simulink model "UV_Model_TT"  (R2020a)
settings: Solver=FixedStepAuto  StartTime=0.0  StopTime=100  FixedStep=0.01  RelTol=1e-3
InitFcn:
  | UV_Parameters;
values from neighbouring files (symbols this model uses):
  KP = 1    [UV_Parameters.m]
  KR = 1    [UV_Parameters.m]
  p0 = [0,0,0]    [UV_Parameters.m]
  R0 = [cos(psi0)*cos(theta0) -sin(psi0)*cos(theta0)+cos(psi0)*sin(theta0)*sin(phi0) sin(psi0)*sin(phi0)+cos(psi0)*sin(theta0)*cos(phi0);        sin(psi0)*cos(theta0) cos(psi0)*cos(theta0)+sin(psi0)*sin(theta0)*sin(phi0)  -cos(psi0)*sin(phi0)+sin(psi0)*sin(theta0)*cos(phi0);        -sin(theta0)  cos(theta0)*sin(phi0)  cos(theta0)*cos(phi0)]    [UV_Parameters.m]
libraries: vrlib x3
settings Model: Creator=vcichella  LastModifiedBy=vcichella
settings SFSimCC: CustomCodeUndefinedFunction=UseInterfaceOnly

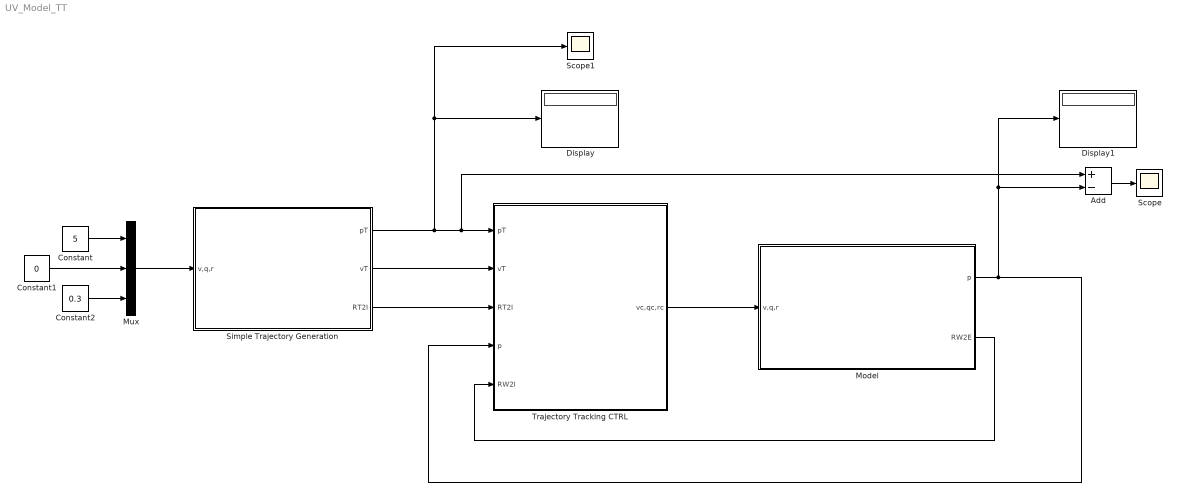
== system UV_Model_TT ==
  Add : Sum  Inputs=+-
  Constant : Constant  Value=5
  Constant1 : Constant  Value=0
  Constant2 : Constant  Value=0.3
  Display : Display
  Display1 : Display
  Model : Subsystem
  Mux : Mux  Inputs=3
  Scope : Scope
  Scope1 : Scope
  Simple Trajectory Generation : Subsystem
  "Trajectory Tracking CTRL " : Subsystem
  wires:
  Simple Trajectory Generation/3(RT2I) -> "Trajectory Tracking CTRL "/3(RT2I)
  Constant/1 -> Mux/1
  Simple Trajectory Generation/1(pT) -> Add/1, "Trajectory Tracking CTRL "/1(pT), Scope1/1, Display/1
  Mux/1 -> Simple Trajectory Generation/1(v,q,r)
  Constant1/1 -> Mux/2
  Constant2/1 -> Mux/3
  Simple Trajectory Generation/2(vT) -> "Trajectory Tracking CTRL "/2(vT)
  Add/1 -> Scope/1
  "Trajectory Tracking CTRL "/1(vc,qc,rc) -> Model/1(v,q,r)
  Model/2(RW2E) -> "Trajectory Tracking CTRL "/5(RW2I)
  Model/1(p) -> "Trajectory Tracking CTRL "/4(p), Add/2, Display1/1

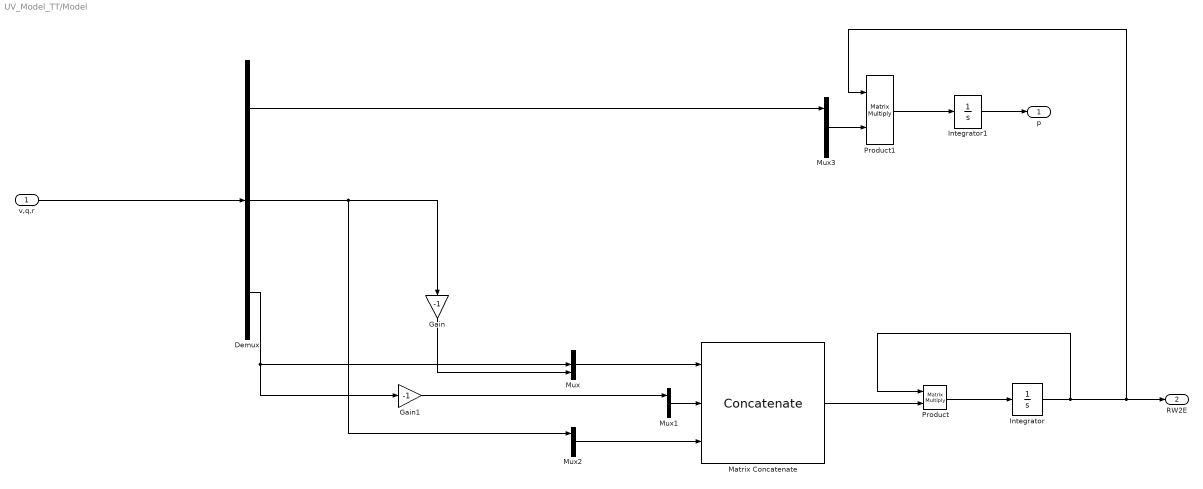
== system UV_Model_TT/Model ==
  v,q,r : Inport
  Demux : Demux  Outputs=3
  Gain : Gain  Gain=-1
  Gain1 : Gain  Gain=-1
  Integrator : Integrator  InitialCondition=R0
  Integrator1 : Integrator  InitialCondition=p0
  Matrix Concatenate : Concatenate  NumInputs=3  Mode=Multidimensional array  ConcatenateDimension=2
  Mux{,1..3} (4 alike) : Mux  Inputs=3
  Product : Product  Multiplication=Matrix(*)
  Product1 : Product  Multiplication=Matrix(*)
  p : Outport  VectorParamsAs1DForOutWhenUnconnected=off
  RW2E : Outport  Port=2  VectorParamsAs1DForOutWhenUnconnected=off
  wires:
  Matrix Concatenate/1 -> Product/2
  v,q,r/1 -> Demux/1
  Mux/1 -> Matrix Concatenate/1
  Demux/3 -> Gain1/1, Mux/2
  Demux/2 -> Mux2/1, Gain/1
  Gain/1 -> Mux/3
  Mux1/1 -> Matrix Concatenate/2
  Gain1/1 -> Mux1/1
  Mux2/1 -> Matrix Concatenate/3
  Product/1 -> Integrator/1
  Integrator1/1 -> p/1
  Product1/1 -> Integrator1/1
  Integrator/1 -> Product1/1, RW2E/1, Product/1
  Mux3/1 -> Product1/2
  Demux/1 -> Mux3/1

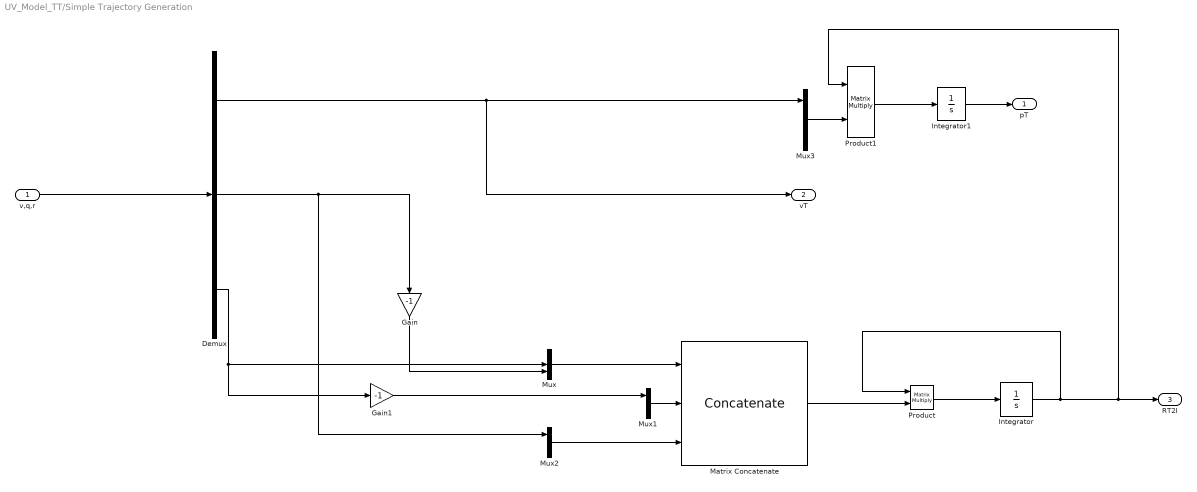
== system UV_Model_TT/Simple Trajectory Generation ==
  v,q,r : Inport
  Demux : Demux  Outputs=3
  Gain : Gain  Gain=-1
  Gain1 : Gain  Gain=-1
  Integrator : Integrator  InitialCondition=R0
  Integrator1 : Integrator  InitialCondition=p0
  Matrix Concatenate : Concatenate  NumInputs=3  Mode=Multidimensional array  ConcatenateDimension=2
  Mux{,1..3} (4 alike) : Mux  Inputs=3
  Product : Product  Multiplication=Matrix(*)
  Product1 : Product  Multiplication=Matrix(*)
  pT : Outport  VectorParamsAs1DForOutWhenUnconnected=off
  vT : Outport  Port=2  VectorParamsAs1DForOutWhenUnconnected=off
  RT2I : Outport  Port=3  VectorParamsAs1DForOutWhenUnconnected=off
  wires:
  Mux3/1 -> Product1/2
  Integrator/1 -> Product/1, RT2I/1, Product1/1
  Product1/1 -> Integrator1/1
  Integrator1/1 -> pT/1
  Demux/1 -> Mux3/1, vT/1
  Product/1 -> Integrator/1
  Mux2/1 -> Matrix Concatenate/3
  Gain1/1 -> Mux1/1
  Mux1/1 -> Matrix Concatenate/2
  Gain/1 -> Mux/3
  Demux/2 -> Gain/1, Mux2/1
  Demux/3 -> Mux/2, Gain1/1
  Mux/1 -> Matrix Concatenate/1
  v,q,r/1 -> Demux/1
  Matrix Concatenate/1 -> Product/2

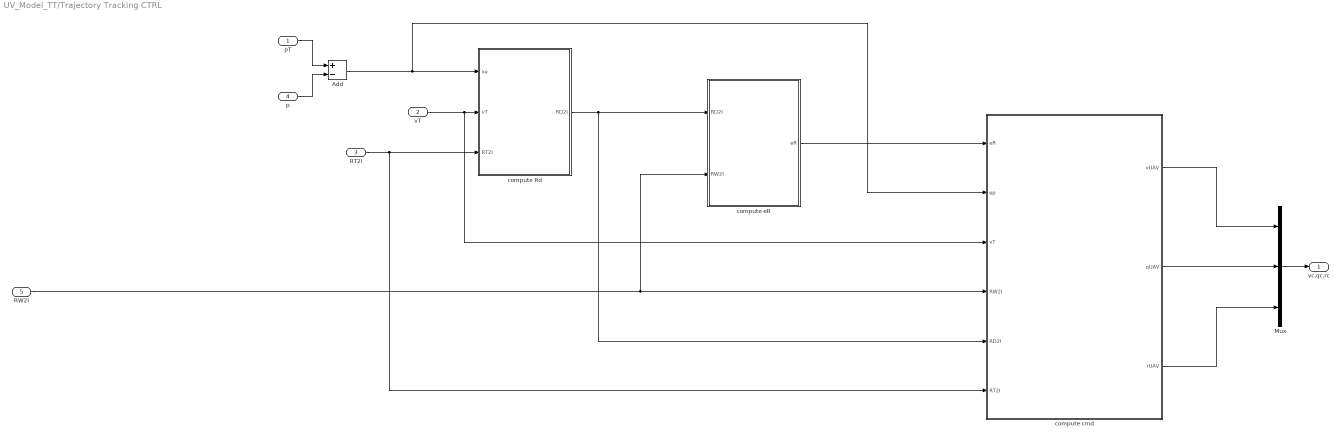
== system UV_Model_TT/Trajectory Tracking CTRL  ==
  pT : Inport
  vT : Inport  Port=2
  RT2I : Inport  Port=3
  p : Inport  Port=4
  RW2I : Inport  Port=5
  Add : Sum  Inputs=+-
  Mux : Mux  Inputs=3
  compute Rd : Subsystem
  compute cmd : Subsystem
  compute eR : Subsystem
  vc,qc,rc : Outport  VectorParamsAs1DForOutWhenUnconnected=off
  wires:
  pT/1 -> Add/1
  p/1 -> Add/2
  vT/1 -> compute cmd/3(vT), compute Rd/2(vT)
  RT2I/1 -> compute cmd/6(RT2I), compute Rd/3(RT2I)
  compute Rd/1(RD2I) -> compute cmd/5(RD2I), compute eR/1(RD2I)
  compute eR/1(eR) -> compute cmd/1(eR)
  Add/1 -> compute cmd/2(ep), compute Rd/1(xe)
  RW2I/1 -> compute eR/2(RW2I), compute cmd/4(RW2I)
  Mux/1 -> vc,qc,rc/1
  compute cmd/1("vUAV ") -> Mux/1
  compute cmd/2(qUAV) -> Mux/2
  compute cmd/3(rUAV) -> Mux/3

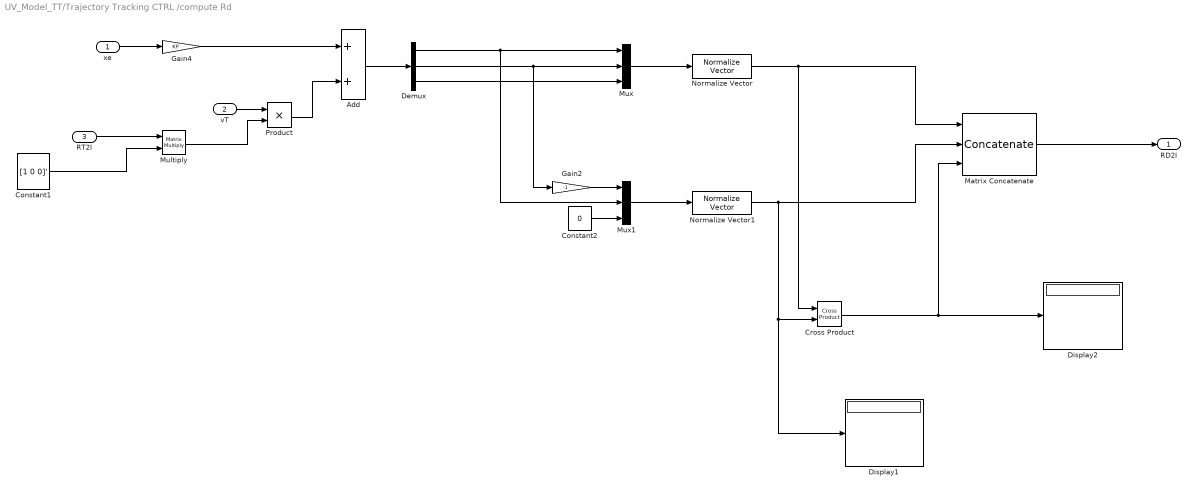
== system UV_Model_TT/Trajectory Tracking CTRL /compute Rd ==
  xe : Inport
  vT : Inport  Port=2
  RT2I : Inport  Port=3
  Add : Sum
  Constant1 : Constant  Value=[1 0 0]'
  Constant2 : Constant  Value=0
  Cross Product : vrlib/Utilities/Cross Product
  Demux : Demux  Outputs=3
  Display1 : Display
  Display2 : Display
  Gain2 : Gain  Gain=-1
  Gain4 : Gain  Gain=KP
  Matrix Concatenate : Concatenate  NumInputs=3  Mode=Multidimensional array  ConcatenateDimension=2
  Multiply : Product  Multiplication=Matrix(*)
  Mux : Mux  Inputs=3
  Mux1 : Mux  Inputs=3
  Normalize Vector : vrlib/Utilities/Normalize Vector  maxzero=0
  Normalize Vector1 : vrlib/Utilities/Normalize Vector  maxzero=0
  Product : Product
  RD2I : Outport  VectorParamsAs1DForOutWhenUnconnected=off
  wires:
  Mux/1 -> Normalize Vector/1
  Demux/3 -> Mux/3
  Mux1/1 -> Normalize Vector1/1
  Normalize Vector/1 -> Cross Product/1, Matrix Concatenate/1
  Normalize Vector1/1 -> Cross Product/2, Display1/1, Matrix Concatenate/2
  Cross Product/1 -> Display2/1, Matrix Concatenate/3
  xe/1 -> Gain4/1
  Matrix Concatenate/1 -> RD2I/1
  vT/1 -> Product/1
  Product/1 -> Add/2
  Add/1 -> Demux/1
  Demux/1 -> Mux1/2, Mux/1
  Constant2/1 -> Mux1/3
  Demux/2 -> Gain2/1, Mux/2
  Multiply/1 -> Product/2
  RT2I/1 -> Multiply/1
  Constant1/1 -> Multiply/2
  Gain4/1 -> Add/1
  Gain2/1 -> Mux1/1

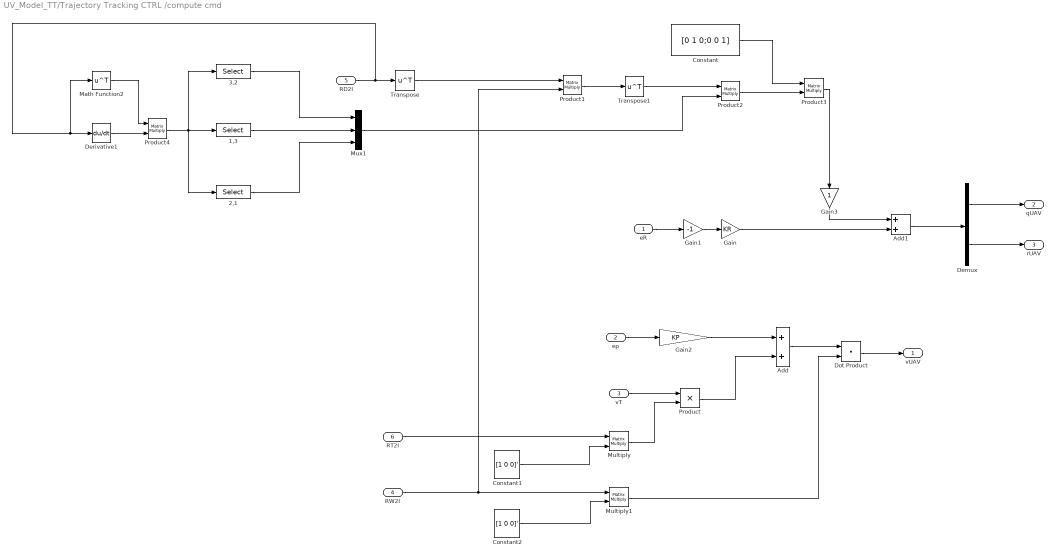
== system UV_Model_TT/Trajectory Tracking CTRL /compute cmd ==
  eR : Inport
  ep : Inport  Port=2
  vT : Inport  Port=3
  RW2I : Inport  Port=4
  RD2I : Inport  Port=5
  RT2I : Inport  Port=6
  1,3 : Selector  NumberOfDimensions=2  InputPortWidth=9  IndexOptions=Index vector (dialog),Index vector (dialog)  Indices=1,3  OutputSizes=1
  2,1 : Selector  NumberOfDimensions=2  InputPortWidth=9  IndexOptions=Index vector (dialog),Index vector (dialog)  Indices=2,1  OutputSizes=1
  3,2 : Selector  NumberOfDimensions=2  InputPortWidth=9  IndexOptions=Index vector (dialog),Index vector (dialog)  Indices=3,2  OutputSizes=1
  Add : Sum
  Add1 : Sum
  Constant : Constant  Value=[0 1 0;0 0 1]
  Constant1 : Constant  Value=[1 0 0]'
  Constant2 : Constant  Value=[1 0 0]'
  Demux : Demux  Outputs=2
  Derivative1 : Derivative
  Dot Product : DotProduct  InputSameDT=on  OutDataTypeStr=Inherit: Inherit via internal rule
  Gain : Gain  Gain=KR
  Gain1 : Gain  Gain=-1
  Gain2 : Gain  Gain=KP
  Gain3 : Gain
  Math Function2 : Math  Operator=transpose  SignedPower=on  SaturateOnIntegerOverflow=on
  Multiply : Product  Multiplication=Matrix(*)
  Multiply1 : Product  Multiplication=Matrix(*)
  Mux1 : Mux  Inputs=3
  Product : Product
  Product1 : Product  Multiplication=Matrix(*)
  Product2 : Product  Multiplication=Matrix(*)
  Product3 : Product  Multiplication=Matrix(*)
  Product4 : Product  Multiplication=Matrix(*)  RndMeth=Zero
  Transpose : Math  Operator=transpose  SignedPower=on  SaturateOnIntegerOverflow=on
  Transpose1 : Math  Operator=transpose  SignedPower=on  SaturateOnIntegerOverflow=on
  "vUAV " : Outport  VectorParamsAs1DForOutWhenUnconnected=off
  qUAV : Outport  Port=2  VectorParamsAs1DForOutWhenUnconnected=off
  rUAV : Outport  Port=3  VectorParamsAs1DForOutWhenUnconnected=off
  wires:
  eR/1 -> Gain1/1
  Gain1/1 -> Gain/1
  Demux/1 -> qUAV/1
  Demux/2 -> rUAV/1
  ep/1 -> Gain2/1
  vT/1 -> Product/1
  Multiply/1 -> Product/2
  Add/1 -> Dot Product/1
  Dot Product/1 -> "vUAV "/1
  Multiply1/1 -> Dot Product/2
  Gain/1 -> Add1/2
  Add1/1 -> Demux/1
  RT2I/1 -> Multiply/1
  Constant1/1 -> Multiply/2
  RW2I/1 -> Product1/2, Multiply1/1
  Constant2/1 -> Multiply1/2
  Transpose/1 -> Product1/1
  Product1/1 -> Transpose1/1
  Transpose1/1 -> Product2/1
  Product2/1 -> Product3/2
  Constant/1 -> Product3/1
  Product3/1 -> Gain3/1
  Gain3/1 -> Add1/1
  Math Function2/1 -> Product4/1
  Mux1/1 -> Product2/2
  2,1/1 -> Mux1/3
  1,3/1 -> Mux1/2
  RD2I/1 -> Derivative1/1, Math Function2/1, Transpose/1
  Product4/1 -> 1,3/1, 3,2/1, 2,1/1
  3,2/1 -> Mux1/1
  Derivative1/1 -> Product4/2
  Product/1 -> Add/2
  Gain2/1 -> Add/1

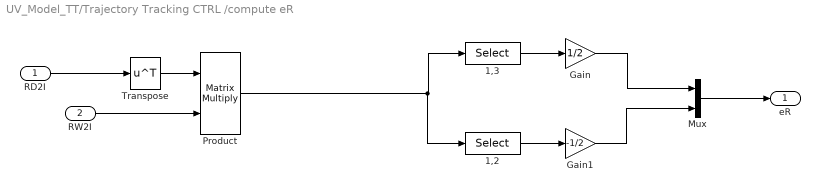
== system UV_Model_TT/Trajectory Tracking CTRL /compute eR ==
  RD2I : Inport
  RW2I : Inport  Port=2
  1,2 : Selector  NumberOfDimensions=2  InputPortWidth=9  IndexOptions=Index vector (dialog),Index vector (dialog)  Indices=1,2  OutputSizes=1
  1,3 : Selector  NumberOfDimensions=2  InputPortWidth=9  IndexOptions=Index vector (dialog),Index vector (dialog)  Indices=1,3  OutputSizes=1
  Gain : Gain  Gain=1/2
  Gain1 : Gain  Gain=-1/2
  Mux : Mux  Inputs=2
  Product : Product  Multiplication=Matrix(*)
  Transpose : Math  Operator=transpose  SignedPower=on  SaturateOnIntegerOverflow=on
  eR : Outport  VectorParamsAs1DForOutWhenUnconnected=off
  wires:
  RD2I/1 -> Transpose/1
  RW2I/1 -> Product/2
  Transpose/1 -> Product/1
  1,3/1 -> Gain/1
  1,2/1 -> Gain1/1
  Mux/1 -> eR/1
  Gain/1 -> Mux/1
  Gain1/1 -> Mux/2
  Product/1 -> 1,2/1, 1,3/1
